simulink model "simscape_earth"  (R2022a)
settings: Solver=ode4  StartTime=0.0  StopTime=12000  FixedStep=1  RelTol=1e-3
undefined symbols (not defined in the file or in its folder): X, Y, Z
libraries: sm_lib x6, nesl_utility x4
settings Model: Creator=sakur  LastModifiedBy=sakur

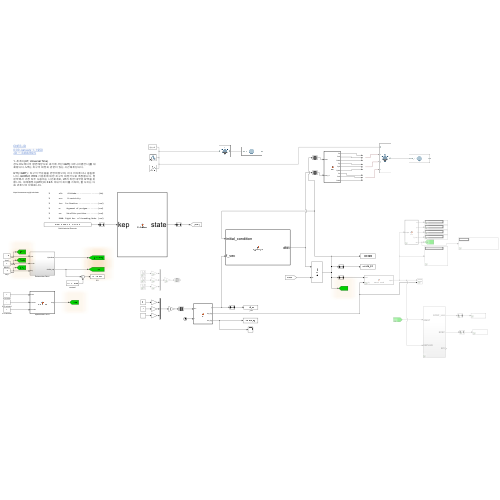
[thumbnail: Simulink's stored preview of the top-level diagram]
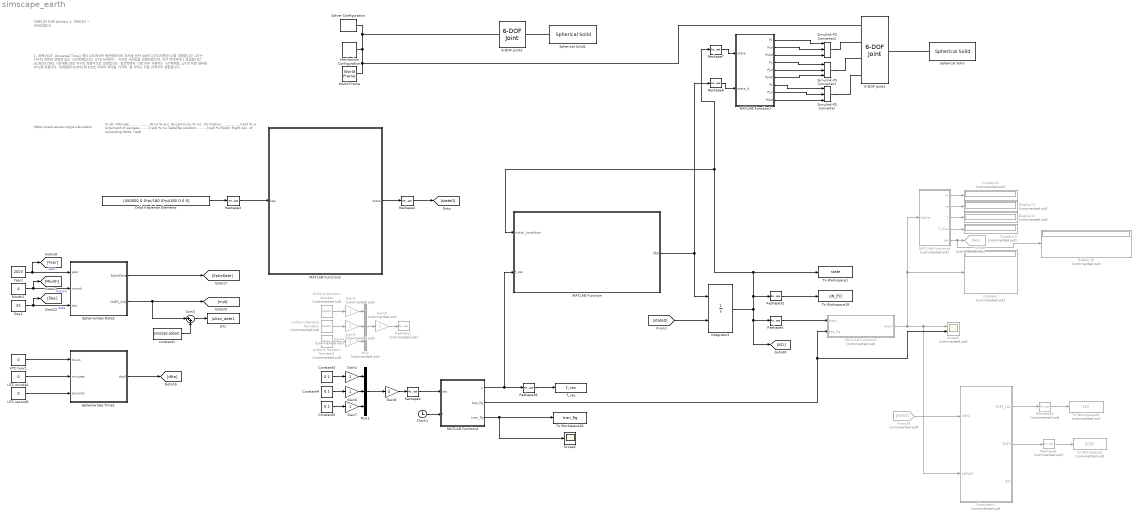
== system simscape_earth ==
  note: % alt: Altitude.....................(Km)
      | % ecc: Eccentricity
      | % inc: Inclination...................(rad)
      | % w: Argument of perigee..........(rad)
      | % nu: Satellite position...........(rad) % RAAN: Right Asc. of Ascending Node. (rad)
  note: 1. 세계시(UT, Universal Time)
      | 경도 0도에서의 평균태양시로 과거에 쓰던 GMT(그리니치평균시)를 대체합니다. UT는 지구의 회전과 관련이 있는 시간체계입니다.
      |
      | UT1(=GMT) : 지구의 극운동을 반영하였으며, 지구 어디에서나 동일합니다. GCRS와 ITRS 기준계에 대한 지구의 회전각으로 측정합니다. 천문학에서 가장 자주 사용하는 시간체계로, UT라 하면 대부분 UT1을 뜻합니다. 세계협정시(UTC)와 0.9초 이내의 차이를 가지며, 둘 사이는 다음 관계식이 성립됩니다.
  note: CNES JD
      | 0:00 January 1, 1950
      | JD − 2433282.5
  note: https://www.aavso.org/jd-calculator
  6-DOF Joint1 : sm_lib/Joints/6-DOF Joint  JointMode=Normal  SenseConstraintForce=off  SenseConstraintForceX=off  SenseConstraintForceY=off  SenseConstraintForceZ=off  SenseConstraintTorque=off  SenseConstraintTorqueX=off  SenseConstraintTorqueY=off  SenseConstraintTorqueZ=off  SenseTotalForce=off  SenseTotalForceX=off  SenseTotalForceY=off  SenseTotalForceZ=off  SenseTotalTorque=off  SenseTotalTorqueX=off  SenseTotalTorqueY=off  SenseTotalTorqueZ=off  CompositeWrenchDir=FollowerOnBase  CompositeWrenchFrame=BaseFrame  PxEquilibriumPosition=0  PxEquilibriumPositionUnits=m  PxSpringStiffness=0  PxSpringStiffnessUnits=N/m  PxDampingCoefficient=0  PxDampingCoefficientUnits=N/(m/s)  PxTorqueActuationMode=ComputedTorque  PxMotionActuationMode=InputMotion  PxSensePosition=off  PxSenseVelocity=off  PxSenseAcceleration=off  PxSenseTorqueForce=off  PxSenseLowerLimitTorqueForce=off  PxSenseUpperLimitTorqueForce=off  PxLowerLimitSpecify=off  PxLowerLimitBound=-1  PxLowerLimitBoundUnits=m  PxLowerLimitStiffness=1e6  PxLowerLimitStiffnessUnits=N/m  PxLowerLimitDamping=1e3  PxLowerLimitDampingUnits=N/(m/s)  PxLowerLimitTransitionRegionWidth=1e-4  PxLowerLimitTransitionRegionWidthUnits=m  PxUpperLimitSpecify=off  PxUpperLimitBound=1  PxUpperLimitBoundUnits=m  PxUpperLimitStiffness=1e6  PxUpperLimitStiffnessUnits=N/m  PxUpperLimitDamping=1e3  PxUpperLimitDampingUnits=N/(m/s)  PxUpperLimitTransitionRegionWidth=1e-4  PxUpperLimitTransitionRegionWidthUnits=m  PxPositionTargetSpecify=off  PxPositionTargetPriority=High  PxPositionTargetValue=0  PxPositionTargetValueUnits=m  PxVelocityTargetSpecify=off  PxVelocityTargetPriority=High  PxVelocityTargetValue=0  PxVelocityTargetValueUnits=m/s  PyEquilibriumPosition=0  PyEquilibriumPositionUnits=m  PySpringStiffness=0  PySpringStiffnessUnits=N/m  PyDampingCoefficient=0  PyDampingCoefficientUnits=N/(m/s)  PyTorqueActuationMode=ComputedTorque  PyMotionActuationMode=InputMotion  PySensePosition=off  PySenseVelocity=off  PySenseAcceleration=off  PySenseTorqueForce=off  PySenseLowerLimitTorqueForce=off  PySenseUpperLimitTorqueForce=off  PyLowerLimitSpecify=off  PyLowerLimitBound=-1  PyLowerLimitBoundUnits=m  PyLowerLimitStiffness=1e6  PyLowerLimitStiffnessUnits=N/m  PyLowerLimitDamping=1e3  PyLowerLimitDampingUnits=N/(m/s)  PyLowerLimitTransitionRegionWidth=1e-4  PyLowerLimitTransitionRegionWidthUnits=m  PyUpperLimitSpecify=off  PyUpperLimitBound=1  PyUpperLimitBoundUnits=m  PyUpperLimitStiffness=1e6  PyUpperLimitStiffnessUnits=N/m  PyUpperLimitDamping=1e3  PyUpperLimitDampingUnits=N/(m/s)  PyUpperLimitTransitionRegionWidth=1e-4  PyUpperLimitTransitionRegionWidthUnits=m  PyPositionTargetSpecify=off  PyPositionTargetPriority=High  PyPositionTargetValue=0  PyPositionTargetValueUnits=m  PyVelocityTargetSpecify=off  PyVelocityTargetPriority=High  PyVelocityTargetValue=0  PyVelocityTargetValueUnits=m/s  PzEquilibriumPosition=0  PzEquilibriumPositionUnits=m  PzSpringStiffness=0  PzSpringStiffnessUnits=N/m  PzDampingCoefficient=0  PzDampingCoefficientUnits=N/(m/s)  PzTorqueActuationMode=ComputedTorque  PzMotionActuationMode=InputMotion  PzSensePosition=off  PzSenseVelocity=off  PzSenseAcceleration=off  PzSenseTorqueForce=off  PzSenseLowerLimitTorqueForce=off  PzSenseUpperLimitTorqueForce=off  PzLowerLimitSpecify=off  PzLowerLimitBound=-1  PzLowerLimitBoundUnits=m  PzLowerLimitStiffness=1e6  PzLowerLimitStiffnessUnits=N/m  PzLowerLimitDamping=1e3  PzLowerLimitDampingUnits=N/(m/s)  PzLowerLimitTransitionRegionWidth=1e-4  PzLowerLimitTransitionRegionWidthUnits=m  PzUpperLimitSpecify=off  PzUpperLimitBound=1  PzUpperLimitBoundUnits=m  PzUpperLimitStiffness=1e6  PzUpperLimitStiffnessUnits=N/m  PzUpperLimitDamping=1e3  PzUpperLimitDampingUnits=N/(m/s)  PzUpperLimitTransitionRegionWidth=1e-4  PzUpperLimitTransitionRegionWidthUnits=m  PzPositionTargetSpecify=off  PzPositionTargetPriority=High  PzPositionTargetValue=0  PzPositionTargetValueUnits=m  PzVelocityTargetSpecify=off  PzVelocityTargetPriority=High  PzVelocityTargetValue=0  PzVelocityTargetValueUnits=m/s  SphDefPosRotationMethod=None  SphDefPosRotationAngleUnits=deg  SphDefPosRotationStandardAxis=+Z  SphDefPosRotationAngle=0.0  SphDefPosRotationArbitraryAxis=[0 0 1]  SphDefPosFollAlignAxisA=+X  SphDefPosBaseAlignAxisA=+Y  SphDefPosFollAlignAxisB=+Y  SphDefPosBaseAlignAxisB=+Z  SphDefPosRotationSequenceAxes=FollowerAxes  SphDefPosRotationSequence=XYX  SphDefPosRotationSequenceAngles=[0 0 0]  SphDefPosRotationSequenceAnglesUnits=deg  SphDefPosRotationMatrix=[1 0 0; 0 1 0; 0 0 1]  SphEqPosRotationMethod=None  SphEqPosRotationAngleUnits=deg  SphEqPosRotationStandardAxis=+Z  SphEqPosRotationAngle=0.0  SphEqPosRotationArbitraryAxis=[0 0 1]  SphEqPosFollAlignAxisA=+X  SphEqPosBaseAlignAxisA=+Y  SphEqPosFollAlignAxisB=+Y  SphEqPosBaseAlignAxisB=+Z  SphEqPosRotationSequenceAxes=FollowerAxes  SphEqPosRotationSequence=XYX  SphEqPosRotationSequenceAngles=[0 0 0]  SphEqPosRotationSequenceAnglesUnits=deg  SphEqPosRotationMatrix=[1 0 0; 0 1 0; 0 0 1]  SphSpringStiffness=0  SphSpringStiffnessUnits=N*m/deg  SphDampingCoefficient=0  SphDampingCoefficientUnits=N*m/(deg/s)  SphActuateTorqueX=off  SphActuateTorqueY=off  SphActuateTorqueZ=off  SphActuateTorque=off  SphTorqueActuationMode=NoTorque  SphMotionActuationMode=ComputedMotion  SphActuationFrame=BaseFrame  SphSensePosition=off  SphSenseVelocityX=off  SphSenseVelocityY=off  SphSenseVelocityZ=off  SphSenseVelocity=off  SphSenseAccelerationX=off  SphSenseAccelerationY=off  SphSenseAccelerationZ=off  SphSenseAcceleration=off  SphSenseTorqueX=off  SphSenseTorqueY=off  SphSenseTorqueZ=off  SphSenseTorqueForce=off  SphSenseLowerLimitTorqueMag=off  SphSenseUpperLimitTorqueMag=off  SphSensingFrame=BaseFrame  SphLowerLimitSpecify=off  SphLowerLimitBound=15  SphLowerLimitBoundUnits=deg  SphLowerLimitStiffness=1e4  SphLowerLimitStiffnessUnits=N*m/deg  SphLowerLimitDamping=10  SphLowerLimitDampingUnits=N*m/(deg/s)  SphLowerLimitTransitionRegionWidth=0.1  SphLowerLimitTransitionRegionWidthUnits=deg  SphUpperLimitSpecify=off  SphUpperLimitBound=45  SphUpperLimitBoundUnits=deg  SphUpperLimitStiffness=1e4  SphUpperLimitStiffnessUnits=N*m/deg  SphUpperLimitDamping=10  SphUpperLimitDampingUnits=N*m/(deg/s)  SphUpperLimitTransitionRegionWidth=0.1  SphUpperLimitTransitionRegionWidthUnits=deg  SphPositionTargetRotationMethod=None  SphPositionTargetRotationAngleUnits=deg  SphPositionTargetRotationStandardAxis=+Z  SphPositionTargetRotationAngle=0.0  SphPositionTargetRotationArbitraryAxis=[0 0 1]  SphPositionTargetFollAlignAxisA=+X  SphPositionTargetBaseAlignAxisA=+Y  SphPositionTargetFollAlignAxisB=+Y  SphPositionTargetBaseAlignAxisB=+Z  SphPositionTargetRotationSequenceAxes=FollowerAxes  SphPositionTargetRotationSequence=XYX  SphPositionTargetRotationSequenceAngles=[0 0 0]  SphPositionTargetRotationSequenceAnglesUnits=deg  SphPositionTargetRotationMatrix=[1 0 0; 0 1 0; 0 0 1]  SphPositionTargetSpecify=off  SphPositionTargetPriority=High  SphVelocityTargetValue=[0 0 0]  SphVelocityTargetValueUnits=deg/s  SphVelocityTargetSpecify=off  SphVelocityTargetPriority=High  SphVelocityTargetInFollowerFrame=on
  6-DOF Joint2 : sm_lib/Joints/6-DOF Joint  JointMode=Normal  SenseConstraintForce=off  SenseConstraintForceX=off  SenseConstraintForceY=off  SenseConstraintForceZ=off  SenseConstraintTorque=off  SenseConstraintTorqueX=off  SenseConstraintTorqueY=off  SenseConstraintTorqueZ=off  SenseTotalForce=off  SenseTotalForceX=off  SenseTotalForceY=off  SenseTotalForceZ=off  SenseTotalTorque=off  SenseTotalTorqueX=off  SenseTotalTorqueY=off  SenseTotalTorqueZ=off  CompositeWrenchDir=FollowerOnBase  CompositeWrenchFrame=BaseFrame  PxEquilibriumPosition=0  PxEquilibriumPositionUnits=m  PxSpringStiffness=0  PxSpringStiffnessUnits=N/m  PxDampingCoefficient=0  PxDampingCoefficientUnits=N/(m/s)  PxTorqueActuationMode=NoTorque  PxMotionActuationMode=ComputedMotion  PxSensePosition=off  PxSenseVelocity=off  PxSenseAcceleration=off  PxSenseTorqueForce=off  PxSenseLowerLimitTorqueForce=off  PxSenseUpperLimitTorqueForce=off  PxLowerLimitSpecify=off  PxLowerLimitBound=-1  PxLowerLimitBoundUnits=m  PxLowerLimitStiffness=1e6  PxLowerLimitStiffnessUnits=N/m  PxLowerLimitDamping=1e3  PxLowerLimitDampingUnits=N/(m/s)  PxLowerLimitTransitionRegionWidth=1e-4  PxLowerLimitTransitionRegionWidthUnits=m  PxUpperLimitSpecify=off  PxUpperLimitBound=1  PxUpperLimitBoundUnits=m  PxUpperLimitStiffness=1e6  PxUpperLimitStiffnessUnits=N/m  PxUpperLimitDamping=1e3  PxUpperLimitDampingUnits=N/(m/s)  PxUpperLimitTransitionRegionWidth=1e-4  PxUpperLimitTransitionRegionWidthUnits=m  PxPositionTargetSpecify=off  PxPositionTargetPriority=High  PxPositionTargetValue=0  PxPositionTargetValueUnits=m  PxVelocityTargetSpecify=off  PxVelocityTargetPriority=High  PxVelocityTargetValue=0  PxVelocityTargetValueUnits=m/s  PyEquilibriumPosition=0  PyEquilibriumPositionUnits=m  PySpringStiffness=0  PySpringStiffnessUnits=N/m  PyDampingCoefficient=0  PyDampingCoefficientUnits=N/(m/s)  PyTorqueActuationMode=NoTorque  PyMotionActuationMode=ComputedMotion  PySensePosition=off  PySenseVelocity=off  PySenseAcceleration=off  PySenseTorqueForce=off  PySenseLowerLimitTorqueForce=off  PySenseUpperLimitTorqueForce=off  PyLowerLimitSpecify=off  PyLowerLimitBound=-1  PyLowerLimitBoundUnits=m  PyLowerLimitStiffness=1e6  PyLowerLimitStiffnessUnits=N/m  PyLowerLimitDamping=1e3  PyLowerLimitDampingUnits=N/(m/s)  PyLowerLimitTransitionRegionWidth=1e-4  PyLowerLimitTransitionRegionWidthUnits=m  PyUpperLimitSpecify=off  PyUpperLimitBound=1  PyUpperLimitBoundUnits=m  PyUpperLimitStiffness=1e6  PyUpperLimitStiffnessUnits=N/m  PyUpperLimitDamping=1e3  PyUpperLimitDampingUnits=N/(m/s)  PyUpperLimitTransitionRegionWidth=1e-4  PyUpperLimitTransitionRegionWidthUnits=m  PyPositionTargetSpecify=off  PyPositionTargetPriority=High  PyPositionTargetValue=0  PyPositionTargetValueUnits=m  PyVelocityTargetSpecify=off  PyVelocityTargetPriority=High  PyVelocityTargetValue=0  PyVelocityTargetValueUnits=m/s  PzEquilibriumPosition=0  PzEquilibriumPositionUnits=m  PzSpringStiffness=0  PzSpringStiffnessUnits=N/m  PzDampingCoefficient=0  PzDampingCoefficientUnits=N/(m/s)  PzTorqueActuationMode=NoTorque  PzMotionActuationMode=ComputedMotion  PzSensePosition=off  PzSenseVelocity=off  PzSenseAcceleration=off  PzSenseTorqueForce=off  PzSenseLowerLimitTorqueForce=off  PzSenseUpperLimitTorqueForce=off  PzLowerLimitSpecify=off  PzLowerLimitBound=-1  PzLowerLimitBoundUnits=m  PzLowerLimitStiffness=1e6  PzLowerLimitStiffnessUnits=N/m  PzLowerLimitDamping=1e3  PzLowerLimitDampingUnits=N/(m/s)  PzLowerLimitTransitionRegionWidth=1e-4  PzLowerLimitTransitionRegionWidthUnits=m  PzUpperLimitSpecify=off  PzUpperLimitBound=1  PzUpperLimitBoundUnits=m  PzUpperLimitStiffness=1e6  PzUpperLimitStiffnessUnits=N/m  PzUpperLimitDamping=1e3  PzUpperLimitDampingUnits=N/(m/s)  PzUpperLimitTransitionRegionWidth=1e-4  PzUpperLimitTransitionRegionWidthUnits=m  PzPositionTargetSpecify=off  PzPositionTargetPriority=High  PzPositionTargetValue=0  PzPositionTargetValueUnits=m  PzVelocityTargetSpecify=off  PzVelocityTargetPriority=High  PzVelocityTargetValue=0  PzVelocityTargetValueUnits=m/s  SphDefPosRotationMethod=None  SphDefPosRotationAngleUnits=deg  SphDefPosRotationStandardAxis=+Z  SphDefPosRotationAngle=0.0  SphDefPosRotationArbitraryAxis=[0 0 1]  SphDefPosFollAlignAxisA=+X  SphDefPosBaseAlignAxisA=+Y  SphDefPosFollAlignAxisB=+Y  SphDefPosBaseAlignAxisB=+Z  SphDefPosRotationSequenceAxes=FollowerAxes  SphDefPosRotationSequence=XYX  SphDefPosRotationSequenceAngles=[0 0 0]  SphDefPosRotationSequenceAnglesUnits=deg  SphDefPosRotationMatrix=[1 0 0; 0 1 0; 0 0 1]  SphEqPosRotationMethod=None  SphEqPosRotationAngleUnits=deg  SphEqPosRotationStandardAxis=+Z  SphEqPosRotationAngle=0.0  SphEqPosRotationArbitraryAxis=[0 0 1]  SphEqPosFollAlignAxisA=+X  SphEqPosBaseAlignAxisA=+Y  SphEqPosFollAlignAxisB=+Y  SphEqPosBaseAlignAxisB=+Z  SphEqPosRotationSequenceAxes=FollowerAxes  SphEqPosRotationSequence=XYX  SphEqPosRotationSequenceAngles=[0 0 0]  SphEqPosRotationSequenceAnglesUnits=deg  SphEqPosRotationMatrix=[1 0 0; 0 1 0; 0 0 1]  SphSpringStiffness=0  SphSpringStiffnessUnits=N*m/deg  SphDampingCoefficient=0  SphDampingCoefficientUnits=N*m/(deg/s)  SphActuateTorqueX=off  SphActuateTorqueY=off  SphActuateTorqueZ=off  SphActuateTorque=off  SphTorqueActuationMode=NoTorque  SphMotionActuationMode=ComputedMotion  SphActuationFrame=BaseFrame  SphSensePosition=off  SphSenseVelocityX=off  SphSenseVelocityY=off  SphSenseVelocityZ=off  SphSenseVelocity=off  SphSenseAccelerationX=off  SphSenseAccelerationY=off  SphSenseAccelerationZ=off  SphSenseAcceleration=off  SphSenseTorqueX=off  SphSenseTorqueY=off  SphSenseTorqueZ=off  SphSenseTorqueForce=off  SphSenseLowerLimitTorqueMag=off  SphSenseUpperLimitTorqueMag=off  SphSensingFrame=BaseFrame  SphLowerLimitSpecify=off  SphLowerLimitBound=15  SphLowerLimitBoundUnits=deg  SphLowerLimitStiffness=1e4  SphLowerLimitStiffnessUnits=N*m/deg  SphLowerLimitDamping=10  SphLowerLimitDampingUnits=N*m/(deg/s)  SphLowerLimitTransitionRegionWidth=0.1  SphLowerLimitTransitionRegionWidthUnits=deg  SphUpperLimitSpecify=off  SphUpperLimitBound=45  SphUpperLimitBoundUnits=deg  SphUpperLimitStiffness=1e4  SphUpperLimitStiffnessUnits=N*m/deg  SphUpperLimitDamping=10  SphUpperLimitDampingUnits=N*m/(deg/s)  SphUpperLimitTransitionRegionWidth=0.1  SphUpperLimitTransitionRegionWidthUnits=deg  SphPositionTargetRotationMethod=None  SphPositionTargetRotationAngleUnits=deg  SphPositionTargetRotationStandardAxis=+Z  SphPositionTargetRotationAngle=0.0  SphPositionTargetRotationArbitraryAxis=[0 0 1]  SphPositionTargetFollAlignAxisA=+X  SphPositionTargetBaseAlignAxisA=+Y  SphPositionTargetFollAlignAxisB=+Y  SphPositionTargetBaseAlignAxisB=+Z  SphPositionTargetRotationSequenceAxes=FollowerAxes  SphPositionTargetRotationSequence=XYX  SphPositionTargetRotationSequenceAngles=[0 0 0]  SphPositionTargetRotationSequenceAnglesUnits=deg  SphPositionTargetRotationMatrix=[1 0 0; 0 1 0; 0 0 1]  SphPositionTargetSpecify=off  SphPositionTargetPriority=High  SphVelocityTargetValue=[0 0 0]  SphVelocityTargetValueUnits=deg/s  SphVelocityTargetSpecify=off  SphVelocityTargetPriority=High  SphVelocityTargetInFollowerFrame=on
  Clock1 : Clock
  Constant3 : Constant  Value=0.1
  Constant4 : Constant  Value=0.1
  Constant5 : Constant  Value=0.1
  Day1 : Constant  Value=25
  Display{1,10..13,19} (6 alike) : Display  Commented=on
  Ephemerides Date1 : Subsystem
  Ephemerides Time1 : MATLAB Function  TreatAsAtomicUnit=on
  From24 : From  Commented=on  GotoTag=GMST
  Gain1 : Gain
  Gain{2..5} (4 alike) : Gain  Commented=on
  Gain6 : Gain
  Gain7 : Gain
  Gain8 : Gain  Gain=0
  Goto8 : Goto  Commented=on  GotoTag=we
  Integrator2 : Integrator  InitialConditionSource=external  InitialCondition=[-7000 0 0 0 -9.175045 0 5233.5]'
  JD1 : ToWorkspace  VariableName=Julian_date1  SampleTime=-1
  MATLAB Function : MATLAB Function  TreatAsAtomicUnit=on
  MATLAB Function1 : MATLAB Function  TreatAsAtomicUnit=on
  MATLAB Function2 : MATLAB Function  TreatAsAtomicUnit=on
  MATLAB Function4 : MATLAB Function  TreatAsAtomicUnit=on
  MATLAB Function5 : MATLAB Function  Commented=on  TreatAsAtomicUnit=on
  MATLAB Function8 : MATLAB Function  Commented=on  TreatAsAtomicUnit=on
  Mechanism Configuration : sm_lib/Utilities/Mechanism Configuration  UniformGravity=None  GravityVector=[0 0 -9.80665]  GravityUnits=m/s^2  LinearizationDelta=0.001  JointModeTransitionNonlinearIterations=2
  Month1 : Constant  Value=4
  Mux : Mux  Commented=on  Inputs=3
  Mux1 : Mux  Inputs=3
  Orbit Keplerian Elements : Constant  Value=[450000 0 0*pi/180 0*pi/180 0 0 0]
  Reshape1 : Reshape  Commented=on  OutputDimensionality=Column vector (2-D)
  Reshape2 : Reshape  OutputDimensionality=Column vector (2-D)
  Reshape{3..5,28,31} (5 alike) : Reshape  OutputDimensionality=Row vector (2-D)
  Reshape32 : Reshape  Commented=on  OutputDimensionality=Row vector (2-D)
  Reshape6 : Reshape  Commented=on  OutputDimensionality=Row vector (2-D)
  Reshape7 : Reshape  OutputDimensionality=Column vector (2-D)
  Reshape8 : Reshape  OutputDimensionality=Column vector (2-D)
  Scope2 : Scope
  Scope5 : Scope  Commented=on  NumInputPorts=2
  Simulink-PS Converter : nesl_utility/Simulink-PS Converter  PhysicalDomain=network_engine_domain  SubClassName=ps_input  LeftPortType=input  RightPortType=output  PseudoPeriodic=off  Frequencies=[]  NoiseDistribution=none  NoiseParameters=[]  Unit=1  AffineConversion=off  FilteringAndDerivatives=provide  SimscapeFilterOrder=1  InputFilterTimeConstant=0.001  UdotUserProvided=2
      settings: SourceProductBaseCode=SS,PW,VE
  Simulink-PS Converter1 : nesl_utility/Simulink-PS Converter  PhysicalDomain=network_engine_domain  SubClassName=ps_input  LeftPortType=input  RightPortType=output  PseudoPeriodic=off  Frequencies=[]  NoiseDistribution=none  NoiseParameters=[]  Unit=1  AffineConversion=off  FilteringAndDerivatives=provide  SimscapeFilterOrder=1  InputFilterTimeConstant=0.001  UdotUserProvided=2
      settings: SourceProductBaseCode=SS,PW,VE
  Simulink-PS Converter2 : nesl_utility/Simulink-PS Converter  PhysicalDomain=network_engine_domain  SubClassName=ps_input  LeftPortType=input  RightPortType=output  PseudoPeriodic=off  Frequencies=[]  NoiseDistribution=none  NoiseParameters=[]  Unit=1  AffineConversion=off  FilteringAndDerivatives=provide  SimscapeFilterOrder=1  InputFilterTimeConstant=0.001  UdotUserProvided=2
      settings: SourceProductBaseCode=SS,PW,VE
  Solver Configuration : nesl_utility/Solver Configuration  PhysicalDomain=network_engine_domain  SubClassName=solver  LeftPortType=input  RightPortType=generic  Tones=[]  Harmonics=[]  SimulateNoise=off  Profile=off  UseLocalSampling=off  EnableSwitchedLinearOptims=on  FrequencyDomain=off  UseCCode=off  RelTol=0.001  AbsTol=0.001  MinStep=1e-09  ToWorkspace=off  RevertToSquareIcSolve=off  NumHomotopyIterations=100  PhasorMode=off  PhasorModeNumHarmonics=1  IndexReductionMethod=DerivativeReplacement  DoDC=off  ResidualTolerance=1e-09  UseLocalSolver=off  LocalSolverChoice=NE_BACKWARD_EULER_ADVANCER  LocalSolverSampleTime=0.001  DoFixedCost=off  MaxNonlinIter=3  MaxModeIter=2  ComputeImpulses=off  ImpulseIterations=2  LinearAlgebra=auto  LinearAlgebraNumThread=0  EquationFormulation=NE_TIME_EF  DelaysMemoryBudget=1024  AutomaticFiltering=on  FilteringTimeConstant=0.001  PartitionStorageMethod=AS_NEEDED  PartitionMemoryBudget=1024  PartitionMethod=ROBUST
      settings: SourceProductBaseCode=SS,PW,VE
  Spherical Solid : sm_lib/Body Elements/Spherical Solid  GraphicAmbientColor=[0.15 0.15 0.15 1.0]  BasedOnType=Mass  CenterOfMass=[0 0 0]  CenterOfMassUnits=m  GraphicDiffuseColor=[1.0 1.0 0.0]  Density=1000  DensityUnits=kg/m^3  DoExposeReferenceFrame=on  GraphicEmissiveColor=[0.0 0.0 0.0 1.0]  ExportEntireGeometry=off  SerializedExposedGeometries=<ExposedGeometries/>  SerializedFrames=<Frames><Frame><Id>Frame1</Id><Value><Name>CoM_F</Name><Origin><Source>CenterOfMassFrame</Source><FeatureName></FeatureName></Origin><PrimaryAxis><DefinedDirection>+Z</DefinedDirection><Source>ReferenceFrame</Source><SourceDirection>+Z</SourceDirection><FeatureName></FeatureName></PrimaryAxis><SecondaryAxis><DefinedDirection>+X</DefinedDirection><Source>ReferenceFrame</Source><SourceDirection>+X</SourceDirection><FeatureName></FeatureName></SecondaryAxis></Value></Frame></Frames>  MarkerShape=Sphere  MarkerSize=10  GraphicType=FromGeometry  InertiaType=CalculateFromGeometry  Mass=5.972*(10^24)  MassUnits=kg  MomentsOfInertia=[1 1 1]  MomentsOfInertiaUnits=kg*m^2  GraphicOpacity=1.0  ProductsOfInertia=[0 0 0]  ProductsOfInertiaUnits=kg*m^2  GraphicShininess=75  GraphicSpecularColor=[0.5 0.5 0.5 1.0]  SphereRadius=100000  SphereRadiusUnits=m  GraphicVisPropType=SimpleVisualProperties
  Spherical Solid1 : sm_lib/Body Elements/Spherical Solid  GraphicAmbientColor=[0.15 0.15 0.15 1.0]  BasedOnType=Mass  CenterOfMass=[0 0 0]  CenterOfMassUnits=m  GraphicDiffuseColor=[0.0 0.6 0.6]  Density=1000  DensityUnits=kg/m^3  DoExposeReferenceFrame=on  GraphicEmissiveColor=[0.0 0.0 0.0 1.0]  ExportEntireGeometry=off  SerializedExposedGeometries=<ExposedGeometries/>  SerializedFrames=<Frames><Frame><Id>Frame1</Id><Value><Name>CoM_F</Name><Origin><Source>CenterOfMassFrame</Source><FeatureName></FeatureName></Origin><PrimaryAxis><DefinedDirection>+Z</DefinedDirection><Source>ReferenceFrame</Source><SourceDirection>+Z</SourceDirection><FeatureName></FeatureName></PrimaryAxis><SecondaryAxis><DefinedDirection>+X</DefinedDirection><Source>ReferenceFrame</Source><SourceDirection>+X</SourceDirection><FeatureName></FeatureName></SecondaryAxis></Value></Frame></Frames>  MarkerShape=Sphere  MarkerSize=10  GraphicType=FromGeometry  InertiaType=CalculateFromGeometry  Mass=5.972*(10^24)  MassUnits=kg  MomentsOfInertia=[1 1 1]  MomentsOfInertiaUnits=kg*m^2  GraphicOpacity=1.0  ProductsOfInertia=[0 0 0]  ProductsOfInertiaUnits=kg*m^2  GraphicShininess=75  GraphicSpecularColor=[0.5 0.5 0.5 1.0]  SphereRadius=6371000  SphereRadiusUnits=m  GraphicVisPropType=AdvancedVisualProperties
  Subsystem1 : Subsystem  Commented=on
  Sum2 : Sum  Inputs=|++
  To Workspace1 : ToWorkspace  VariableName=state  SampleTime=-1
      settings: Save2DSignal=2-D array (concatenate along first dimension)
  To Workspace18 : ToWorkspace  VariableName=tran_flg  SampleTime=-1
      settings: Save2DSignal=2-D array (concatenate along first dimension)
  To Workspace19 : ToWorkspace  VariableName=LIN_ECI  SampleTime=-1
      settings: Save2DSignal=2-D array (concatenate along first dimension)
  To Workspace2 : ToWorkspace  Commented=on  VariableName=ECEF  SampleTime=-1
      settings: Save2DSignal=2-D array (concatenate along first dimension)
  To Workspace20 : ToWorkspace  Commented=on  VariableName=LLA  SampleTime=-1
      settings: Save2DSignal=2-D array (concatenate along first dimension)
  UTC hour1 : Constant  Value=0
  UTC minute1 : Constant  Value=0
  UTC second1 : Constant  Value=0
  Uniform Random Number : UniformRandomNumber  Commented=on  Minimum=-0.5  Maximum=0.5  SampleTime=1
  Uniform Random Number1 : UniformRandomNumber  Commented=on  Minimum=-0.5  Maximum=0.5  SampleTime=1
  Uniform Random Number2 : UniformRandomNumber  Commented=on  Minimum=-0.5  Maximum=0.5  SampleTime=1
  World Frame : sm_lib/Frames and Transforms/World Frame
  Year1 : Constant  Value=2023
  constant1 : Constant  Value=2433282.50000
  f_vec : ToWorkspace  VariableName=f_vec  SampleTime=-1
      settings: Save2DSignal=2-D array (concatenate along first dimension)
  wires:
  Ephemerides Time1/1(dayf) -> [dfra]
  MATLAB Function8/1(ra) -> Display10/1
  Gain8/1 -> Reshape2/1
  MATLAB Function8/3(T) -> Display12/1
  Gain2/1 -> Mux/1
  Reshape28/1 -> f_vec/1
  Orbit Keplerian Elements/1 -> Reshape3/1
  Gain1/1 -> Mux1/1
  UTC second1/1 -> Ephemerides Time1/3(seconds)
  Year1/1 -> Ephemerides Date1/1(year), [Year]  "year"
  MATLAB Function8/2(rp) -> Display11/1
  UTC hour1/1 -> Ephemerides Time1/1(hours)
  MATLAB Function8/4(T_hour) -> Display13/1
  Sum2/1 -> JD1/1
  Gain7/1 -> Mux1/3
  MATLAB Function4/1(y) -> MATLAB Function/2(f_vec), Reshape28/1
  Month1/1 -> [Month], Ephemerides Date1/2(month)  "month"
  Mux1/1 -> Gain8/1
  Clock1/1 -> MATLAB Function4/2(t)
  Gain6/1 -> Mux1/2
  Ephemerides Date1/2(CNES_mdj) -> Sum2/1, [mjd]
  Reshape5/1 -> MATLAB Function5/1(statv)
  Mux/1 -> Gain5/1
  MATLAB Function5/1(kepel) -> MATLAB Function8/1(kepler), Display1/1, Subsystem1/2(KEPLER), Scope5/1
  Uniform Random Number/1 -> Gain2/1
  Uniform Random Number1/1 -> Gain3/1
  MATLAB Function4/3(tran_flg) -> Scope2/1, To Workspace18/1
  Constant5/1 -> Gain7/1
  MATLAB Function2/1(state) -> Reshape4/1
  [state0] -> Integrator2/2
  MATLAB Function/1(dfdt) -> Integrator2/1, Reshape8/1
  Ephemerides Date1/1(EpheDate) -> [EpheDate]
  Reshape3/1 -> MATLAB Function2/1(kep)
  Reshape6/1 -> To Workspace2/1
  Constant3/1 -> Gain1/1
  Reshape31/1 -> To Workspace19/1
  Reshape4/1 -> [state0]
  MATLAB Function4/2(kep_flg) -> Scope5/2, MATLAB Function5/2(kep_flg)
  Uniform Random Number2/1 -> Gain4/1
  UTC minute1/1 -> Ephemerides Time1/2(minutes)
  Gain4/1 -> Mux/3
  Day1/1 -> [Day], Ephemerides Date1/3(day)  "date"
  Gain5/1 -> Reshape1/1
  Subsystem1/2(ECEF) -> Reshape6/1
  constant1/1 -> Sum2/2
  MATLAB Function8/5(we) -> Display19/1, Goto8/1
  From24/1 -> Subsystem1/1(GMST)
  Gain3/1 -> Mux/2
  Reshape2/1 -> MATLAB Function4/1(vec)
  Constant4/1 -> Gain6/1
  Reshape32/1 -> To Workspace20/1
  Subsystem1/1(ECEF_LLA) -> Reshape32/1
  Integrator2/1 -> MATLAB Function/1(initial_condition), Reshape7/1, To Workspace1/1, Reshape31/1, Reshape5/1, [ECI]
  MATLAB Function1/7(Pz) -> Simulink-PS Converter/1
  MATLAB Function1/4(Py) -> Simulink-PS Converter1/1
  MATLAB Function1/1(Px) -> Simulink-PS Converter2/1
  Reshape7/1 -> MATLAB Function1/1(state)
  Reshape8/1 -> MATLAB Function1/2(state_d)
  MATLAB Function1/2(Pxd) -> Simulink-PS Converter2/2
  MATLAB Function1/3(Pxdd) -> Simulink-PS Converter2/3
  MATLAB Function1/5(Pyd) -> Simulink-PS Converter1/2
  MATLAB Function1/6(Pydd) -> Simulink-PS Converter1/3
  MATLAB Function1/8(Pzd) -> Simulink-PS Converter/2
  MATLAB Function1/9(Pzdd) -> Simulink-PS Converter/3
  connections:
  Solver Configuration/RConn1 -- Mechanism Configuration/RConn1 -- 6-DOF Joint1/LConn1 -- World Frame/RConn1 -- 6-DOF Joint2/LConn1
  Spherical Solid/LConn1 -- 6-DOF Joint1/RConn1
  Simulink-PS Converter/RConn1 -- 6-DOF Joint1/LConn4
  Simulink-PS Converter1/RConn1 -- 6-DOF Joint1/LConn3
  Simulink-PS Converter2/RConn1 -- 6-DOF Joint1/LConn2
  Spherical Solid1/LConn1 -- 6-DOF Joint2/RConn1

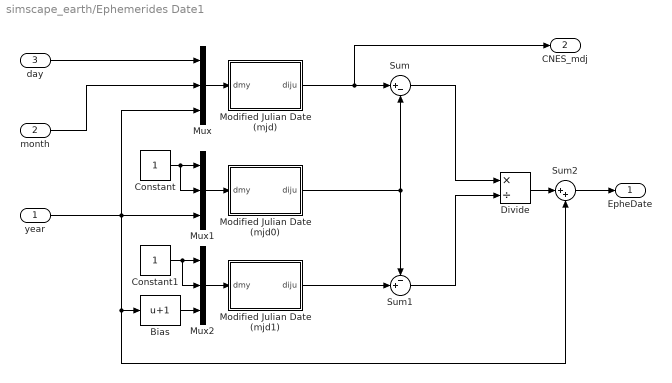
== system simscape_earth/Ephemerides Date1 ==
  year : Inport
  month : Inport  Port=2
  day : Inport  Port=3
  Bias : Bias  Bias=1  SaturateOnIntegerOverflow=off
  Constant : Constant
  Constant1 : Constant
  Divide : Product  Inputs=*/
  Modified Julian Date (mjd) : MATLAB Function  TreatAsAtomicUnit=on
  Modified Julian Date (mjd0) : MATLAB Function  TreatAsAtomicUnit=on
  Modified Julian Date (mjd1) : MATLAB Function  TreatAsAtomicUnit=on
  Mux : Mux  Inputs=3
  Mux1 : Mux  Inputs=3
  Mux2 : Mux  Inputs=3
  Sum : Sum  Inputs=|+-
  Sum1 : Sum  Inputs=-+|
  Sum2 : Sum  Inputs=|++
  EpheDate : Outport
  CNES_mdj : Outport  Port=2
  wires:
  Sum1/1 -> Divide/2
  Modified Julian Date (mjd1)/1(diju) -> Sum1/2
  month/1 -> Mux/2
  year/1 -> Mux1/3, Mux/3, Bias/1, Sum2/2
  Mux1/1 -> Modified Julian Date (mjd0)/1(dmy)
  day/1 -> Mux/1
  Mux/1 -> Modified Julian Date (mjd)/1(dmy)
  Mux2/1 -> Modified Julian Date (mjd1)/1(dmy)
  Bias/1 -> Mux2/3
  Modified Julian Date (mjd)/1(diju) -> CNES_mdj/1, Sum/1
  Constant1/1 -> Mux2/2, Mux2/1
  Sum/1 -> Divide/1
  Constant/1 -> Mux1/2, Mux1/1
  Modified Julian Date (mjd0)/1(diju) -> Sum1/1, Sum/2
  Divide/1 -> Sum2/1
  Sum2/1 -> EpheDate/1

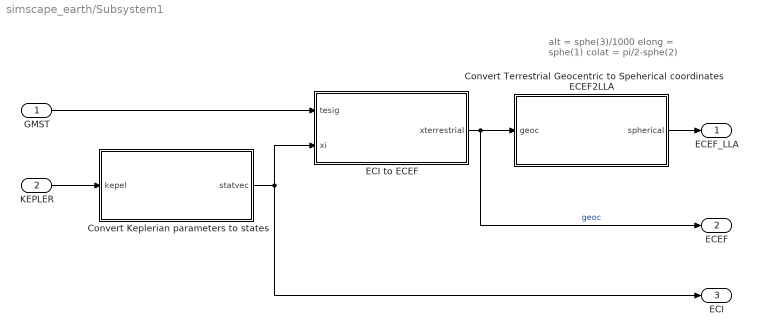
== system simscape_earth/Subsystem1 ==
  note: alt = sphe(3)/1000
      | elong = sphe(1)
      | colat = pi/2-sphe(2)
  GMST : Inport
  KEPLER : Inport  Port=2
  Convert Keplerian parameters to states : MATLAB Function  TreatAsAtomicUnit=on
  Convert Terrestrial Geocentric to Speherical coordinates ECEF2LLA : MATLAB Function  TreatAsAtomicUnit=on
  "ECI to ECEF " : MATLAB Function  TreatAsAtomicUnit=on
  ECEF_LLA : Outport
  ECEF : Outport  Port=2
  ECI : Outport  Port=3
  wires:
  "ECI to ECEF "/1(xterrestrial) -> ECEF/1, Convert Terrestrial Geocentric to Speherical coordinates ECEF2LLA/1(geoc)  "geoc"
  Convert Terrestrial Geocentric to Speherical coordinates ECEF2LLA/1(spherical) -> ECEF_LLA/1
  Convert Keplerian parameters to states/1(statvec) -> "ECI to ECEF "/2(xi), ECI/1
  GMST/1 -> "ECI to ECEF "/1(tesig)
  KEPLER/1 -> Convert Keplerian parameters to states/1(kepel)

== matlab function simscape_earth/Subsystem1/Convert Keplerian parameters to states ==
  data: kepel input; statvec output
function statvec = kepel_statvec(kepel)
%  [statvec] = kepel_statvec (kepel)
%	The function kepel_statvec transforms the keplerian
%	elements kepel into the corresponding state vector in
%	the same reference system.
%
% Input:
%	kepel
% 		vector containing the keplerian elements:
%		(1) - semimajor axis of the orbit in meters.
%		(2) - eccentricity.
%		(3) - inclination in radians.
%		(4) - right ascension of ascending node in radians.
%		(5) - argument of perigee in radians.
%		(6) - mean anomaly in radians.
%
% Output:
%	statvec
%  		state vector in meters and meters/second.
%
% Authors:
%	Helio K. Kuga;
%	Valder M. Medeiros;
%	Valdemir Carrara		february/80		version 1.0
%	Valdemir Carrara		july 2005		(C version)
%   Valdemir Carrara            March/09        Matlab

EARTH_GRAVITY	= 3.9860064e+14;		% Earth's gravitational constant (m**3/s**2)

a    = kepel(1);	% semi-major axis
exc  = kepel(2);	% eccentricity

c1   = sqrt(1. - exc*exc);

% Rotational matrix
rot_maz1 =  [cos(-kepel(4)), sin(-kepel(4)), 0;
             -sin(-kepel(4)), cos(-kepel(4)), 0; 
             0, 0, 1];
         
rot_max =  [1, 0, 0; 
           0, cos(-kepel(3)), sin(-kepel(3));
           0, -sin(-kepel(3)), cos(-kepel(3))];
       
rot_maz2 =  [cos(-kepel(5)), sin(-kepel(5)), 0;
             -sin(-kepel(5)), cos(-kepel(5)), 0; 
             0, 0, 1];
         
orb2iner = rot_maz1*rot_max*rot_maz2;

%%%%%%%%%%%%%%%%%%%%%%%%%%%%%%%%%%%%%%%%%%%%
%     Kepler's equation
%E    = kepler(kepel(6), exc);
mean_anomaly = kepel(6);
eccentricity = exc;
%function [eccentric] = kepler (mean_anomaly, eccentricity)
% [eccentric] = kepler (mean_anomaly, eccentricity)
%	The subroutine kepler finds a solution to the
%	kepler's equation.
%
% Input:
%	mean_anomaly
%		mean anomaly in radians.
%	eccentricity
%		eccentricity.
%
% Output:
%	eccentric
%		eccentric anomaly in radians.
%
% Authors:
%	Valder M. de Medeiros		june/81		version 2.0
%	Valdemir Carrara			july 2005	(C version)
%   Valdemir Carrara            March/09        Matlab

exc2    = eccentricity*eccentricity;
am1     = mod (mean_anomaly, 2*pi);
am2     = am1 + am1;
am3     = am1 + am2;
shoot   = am1 + eccentricity*(1. - 0.125*exc2)*sin(am1) + ...
		0.5*exc2*(sin(am2) + 0.75*eccentricity*sin(am3));
shoot   = mod (shoot, 2*pi);

e1      = 1.0;
ic      = 0;

while ((abs(e1) > 1.e-12) && (ic <= 10)) 
	e1    = (shoot - am1 - eccentricity*sin(shoot)) / ...
			(1.0 - eccentricity*cos(shoot));
    shoot = shoot - e1;
    ic    = ic + 1;
end

if (ic >= 10)
    disp ('warning ** subroutine kepler did not converge in 10 iterations');
end

%eccentric = shoot;
E = shoot;
%%%%%%%%%%%%%%%%%%%%%%%%%%%%%%%%%%%%%%%%%%%%%%
sE   = sin(E);
cE   = cos(E);
c3   = sqrt(EARTH_GRAVITY/a)/(1. - exc*cE);

%     state vector

statvec = [[a*(cE - exc), a*c1*sE, 0]*orb2iner', [-c3*sE, c1*c3*cE, 0]*orb2iner'];

== matlab function simscape_earth/Subsystem1/Convert Terrestrial Geocentric to Speherical coordinates ECEF2LLA ==
  data: geoc input; spherical output
function spherical  = rectangular_to_spherical (geoc)
% [spherical] = rectangular_to_spherical (geoc)
%	Function to transform rectangular terrestrial
%	geocentric coordinates in spherical coordinates
%	(longitude, geocentric latitude and distance).
%
% Inputs:
%   geoc
%   		geocentric rectangular coordinates vector in meters
%           (1) geocentric position x (m)
%           (2) geocentric position y (m)
%           (3) geocentric position z (m)
%
% Outputs:
%	spherical
%		Geocentric coordinates vector:
%			1 = east longitude (rad)
%			2 = geocentric latitude (rad)
%			3 = geocentric distance (meters)
%
% Authors:
%   Valdemir Carrara            May/09        Matlab

px = geoc(1);
py = geoc(2);
pz = geoc(3);
ws = px*px + py*py;
rw = sqrt(ws + pz *pz);
lg = atan2(py, px);
lt = atan2(pz, sqrt(ws));
spherical = [lg, lt, rw];

== matlab function simscape_earth/Subsystem1/ECI to ECEF  ==
  data: tesig input; xterrestrial output; xi input
function xterrestrial  = inertial_to_terrestrial (tesig, xi)
% [xterrestrial] = inertial_to_terrestrial (tesig, xi)
%	The function inertial_to_terrestrial transforms geocentric
%	inertial state vector into geocentric
%	terrestrial coordinates (referred to
%	Greenwich).
%
% Input:
%	tesig
%		Greenwich sidereal time in radians.
%	xi
%		geocentric inertial position vector.
%       (1) inertial geocentric position x (m)
%       (2) inertial geocentric position y (m)
%       (3) inertial geocentric position z (m)
%       (4) inertial geocentric velocity x (m/s)
%       (5) inertial geocentric velocity y (m/s)
%       (6) inertial geocentric velocity z (m/s)
%
% Output:
%	xterrestrial
%		corresponding geocentric terrestrial vector.
%
% Authors:
%	Helio/Valder/Valdemir-aug. 1981 - version 1.0
%	Helio		-july 1989 - version 1.1
%	Valdemir Carrara		july 2005		(C version)
%   Valdemir Carrara            March/09        Matlab
coan    =  cos(tesig);
sian    =  sin(tesig);
rot_mat =  [ coan, sian, 0 ;
            -sian, coan, 0 ; 
                0,    0, 1];

xterrestrial_ = [xi(1:3); xi(4:6)]*rot_mat';
xterrestrial  = [xterrestrial_(1,:) xterrestrial_(2,:)];

== matlab function simscape_earth/MATLAB Function1 ==
  data: state input; Px output; Pxd output; Pxdd output; state_d input; Py output; Pyd output; Pydd output; Pz output; Pzd output; Pzdd output
function [Px,Pxd,Pxdd,Py,Pyd,Pydd,Pz,Pzd,Pzdd] = fcn(state, state_d)
Px   = state(1,1);
Py   = state(2,1);
Pz   = state(3,1);
Pxd  = state(4,1);
Pyd  = state(5,1);
Pzd  = state(6,1);
Pxdd = state_d(4,1);
Pydd = state_d(5,1);
Pzdd = state_d(6,1);
end

== matlab function simscape_earth/MATLAB Function ==
  data: initial_condition input; dfdt output; f_vec input
function dfdt  = eq_propagate(initial_condition, f_vec)
% u=3.9865*10^14;
u=3.9865*10^14;
% Re=6378.14;         % Earth Radius
Re = 6378137; % earth radius in m

dfdt = zeros(size(initial_condition));

%x=x
%x1=dx/dt
%dx1/dt = d^2(x)/dt
% f_vec = [rand(1)*0 rand(1)*0 rand(1)*0]';

x1 = initial_condition(4); % x1 = dx/dt
y1 = initial_condition(5); % y1 = dy/dt
z1 = initial_condition(6); % z1 = dz/dt
x  = initial_condition(1); % x
y  = initial_condition(2); % y
z  = initial_condition(3); % z

m  = initial_condition(7); % mass

r=sqrt(x^2+y^2+z^2);

% % %   Keplar Motion Equatnion
% % %  => r_dd + u/(r^3)r_ = 0 => r_dd = -u/(r^3)r_
dfdt(1) = x1;
dfdt(2) = y1;
dfdt(3) = z1;
dfdt(4) = -u*x/r^3 + f_vec(1,1);
dfdt(5) = -u*y/r^3 + f_vec(2,1);
dfdt(6) = -u*z/r^3 + f_vec(3,1);
dfdt(7) = 0;
end

== matlab function simscape_earth/MATLAB Function2 ==
  data: kep input; state output
% function [X, Y, Z, Vx, Vy, Vz] = Kepler2Carts(alt, ecc, inc, w, nu, RAAN)
function state = Kepler2Carts(kep)
%--------------------------------------------------------------------------------------------------------%
%
% 			USAGE: Conversion of Keplerian Classic Orbital Elements into geocentric-equatorial reference system OXYZ
%
% 			AUTHOR: Thameur Chebbi(PhD)		E-MAIL: chebbythamer@gmail.com
%
% 			DATE: 01,Oct,2020
%
% 			DESCIPTION:      This function is created to convert the classical 
%               		     orbital elements to cartesian position and velocity 
%		       		         parameters of any satellite orbit in the geocentric-equatorial
%                            reference system.
%
% 			INPUT:
%           kep0 =>
% 			alt:    Altitude.....................(Km)							
% 			ecc:    Eccentricity											    
% 			inc:	Inclination..................(rad)							
% 			w:	    Argument of perigee..........(rad)	
% 			nu:	    Satellite position...........(rad)							
% 			RAAN:	Right Asc. of Ascending Node.(rad)							
%
% 			OUTPUT:
%			Position Components: 		
% 			[X  Y  Z ]....(Km)
%
%			Velocity Components:
% 			[Vx Vy Vz]....(Km/s) 														
%
alt  = kep(1,1);    ecc  = kep(1,2);
inc  = kep(1,3);    w    = kep(1,4);
nu   = kep(1,5);    RAAN = kep(1,6);
%%---------------------------- Constants ----------------------------------------------%
% mu_earth = 3.986 * 10^5; % Earth Gravitational Constant
mu_earth = 3.9865 * 10^14; % Earth Gravitational Constant
% re = 6378.1; % earth radius in km
re = 6378137; % earth radius in m
%
%%--------------------------------------------------------------------------------------
a = alt + re;
p = a*(1-ecc ^2);
r_0 = p / (1 + ecc * cos(nu));
%
%%--------------- Coordinates in the perifocal reference system Oxyz -----------------%
%
% position vector coordinates
x = r_0 * cos(nu);
y = r_0 * sin(nu);
%
%
% velocity vector coordinates
Vx_ = -(mu_earth/p)^(1/2) * sin(nu);
Vy_ = (mu_earth/p)^(1/2) * (ecc + cos(nu));
%
%
%%-------------- the geocentric-equatorial reference system OXYZ ---------------------%
%
% position vector components X, Y, and Z
X = (cos(RAAN) * cos(w) - sin(RAAN) * sin(w) * cos(inc)) * x + (-cos(RAAN) * sin(w) - sin(RAAN) * cos(w) * cos(inc)) * y;
Y = (sin(RAAN) * cos(w) + cos(RAAN) * sin(w) * cos(inc)) * x + (-sin(RAAN) * sin(w) + cos(RAAN) * cos(w) * cos(inc)) * y;
Z = (sin(w) * sin(inc)) * x + (cos(w) * sin(inc)) * y;
% velocity vector components X', Y', and Z'
Vx = (cos(RAAN) * cos(w) - sin(RAAN) * sin(w) * cos(inc)) * Vx_ + (-cos(RAAN) * sin(w) - sin(RAAN) * cos(w) * cos(inc)) * Vy_;
Vy = (sin(RAAN) * cos(w) + cos(RAAN) * sin(w) * cos(inc)) * Vx_ + (-sin(RAAN) * sin(w) + cos(RAAN) * cos(w) * cos(inc)) * Vy_;
Vz = (sin(w) * sin(inc)) * Vx_ + (cos(w) * sin(inc)) * Vy_;

state = [X,Y,Z,Vx,Vy,Vz,10];

end

== matlab function simscape_earth/MATLAB Function4 ==
  settings: updateMethod=DISCRETE
  data: vec input; y output; kep_flg output; t input; tran_flg output
function [y, kep_flg, tran_flg] = fcn(vec, t)
ft = 10000;
dt = 1000;


persistent first_flg
persistent tran_flg_save


if isempty(first_flg)
    tran_flg_save = 0;
    first_flg = 1;
end

if tran_flg_save == 0
    if( t <= ft )
        y = 0*vec;
    else
        tran_flg_save = tran_flg_save + 1;
        y = 0*vec;
    end
    kep_flg  = 1;

elseif tran_flg_save == 1
    if ((t>ft) && (t<=(ft+dt)))%firing
        y = 1*vec;
        kep_flg  = 0;
    else
        y = 0*vec;
        kep_flg  = 1;
        tran_flg_save = tran_flg_save + 1;
    end

elseif tran_flg_save == 2
    y = 0*vec;
    kep_flg  = 1;
else
    y = 0*vec;
    kep_flg  = 1;
end

tran_flg = tran_flg_save;

% if ((t>=ft) && (t<=(ft+dt)))
%     y = 1*vec;
%     kep_flg  = 0;
%     tran_flg = 1;
% else
%     y = 0*vec;
%     kep_flg  = 1;
%     tran_flg_save = 0;
% end

end

== matlab function simscape_earth/MATLAB Function5 ==
  settings: updateMethod=DISCRETE
  data: statv input; kepel output; kep_flg input
function kepel  = statvec_kepel (statv, kep_flg)
%	The function statvec_kepel transforms the state vector statv
%	into the corresponding keplerian elements in the
%	same reference system.
%
% Input:
%	statv
%		state vector in meters and meters/second.
%
% Output:
%	statvec_kepel
%		vector containing the keplerian elements:
%		(1) - semimajor axis of the orbit in meters.
%		(2) - eccentricity.
%		(3) - inclination in radians.
%		(4) - right ascension of ascending node in radians.
%		(5) - argument of perigee in radians.
%		(6) - mean anomaly in radians.
persistent kepel_save
persistent first_flg

if isempty(first_flg)
    kepel_save = [0 0 0 0 0 0];
    first_flg = 1;
end

EARTH_GRAVITY	= 3.9860064e+14;		% Earth's gravitational constant (m**3/s**2)

if kep_flg == 1
    xp     = [statv(1),statv(2),statv(3)];
    xv     = [statv(4),statv(5),statv(6)];
    r      = sqrt(xp*xp');
    vq     = xv*xv';
    ainv   = 2.0/(r) - vq/EARTH_GRAVITY;

    h      = cross(xp, xv);
    hm     = sqrt(h*h');
    if (hm < 1.e-10)
        disp (' *** Message from function statvec_kepel: *** ');
        disp (' There are no keplerian elements corresponding to this state vector');
        kepel = [0, 0, 0, 0, 0, 0];
    else
        h      = h/hm;
        incl   = acos(h(3));
        raan   = atan2(h(1), -h(2));
        d      = xp*xv' / EARTH_GRAVITY;
        esene  = d * sqrt(EARTH_GRAVITY*ainv);
        ecose  = 1 - r*ainv;
        exc    = sqrt(esene*esene + ecose*ecose);
        E      = atan2(esene, ecose);
        mean   = mod (E - esene, 2*pi);
        an = [0 0 0];
        if mean < 0
            mean = mean + 2*pi;
        end
        if exc < 1.e-10
            arpe = 0;
        else
            dp     = 1./r - ainv;
            ev     = dp*xp - d*xv;
            abev   = sqrt(ev*ev');
            ev     = ev/abev;
            an(1)  = cos(raan);
            an(2)  = sin(raan);
            an(3)  = 0;
            fi     = ev*cross(h, an)';
            arpe = acos(ev*an');
            if fi < 0
                arpe  =  -arpe + 2*pi;
            end
        end

        kepel = [(1./ainv), exc, incl, raan, arpe, mean];
        kepel_save = kepel;
%         T = 2*pi*sqrt((a*a*a)/(EARTH_GRAVITY));
    end
else

    kepel = kepel_save;
    T = 0;
end


end

== matlab function simscape_earth/Ephemerides Date1/Modified Julian Date (mjd) ==
  data: dmy input; diju output
function diju  =  djm (dmy)
% [diju] = djm (day, month, year)
%    The function djm furnishes the Modified Julian
%    Date with reference to the day, month and year,
%    at zero hours of the day.
% inputs:
%   dmy(1): day, day of the month
%   dmy(2): month, month of the year
%   dmy(3): year

% outputs:
%   diju
%       Modified Julian Date in days, referred to 1950.0. 
%
% Valdemir Carrara, Apr, 2003
%

diju = 367*dmy(3) + dmy(1) - 712269 + fix(275*dmy(2)/9)- fix(7*(dmy(3)+fix((dmy(2)+9)/12))/4);

== matlab function simscape_earth/Ephemerides Date1/Modified Julian Date (mjd0) ==
  data: dmy input; diju output
function diju  =  djm (dmy)
% [diju] = djm (day, month, year)
%    The function djm furnishes the Modified Julian
%    Date with reference to the day, month and year,
%    at zero hours of the day.
% inputs:
%   dmy(1): day, day of the month
%   dmy(2): month, month of the year
%   dmy(3): year

% outputs:
%   diju
%       Modified Julian Date in days, referred to 1950.0. 
%
% Valdemir Carrara, Apr, 2003
%

diju = 367*dmy(3) + dmy(1) - 712269 + fix(275*dmy(2)/9)- fix(7*(dmy(3)+fix((dmy(2)+9)/12))/4);

== matlab function simscape_earth/Ephemerides Date1/Modified Julian Date (mjd1) ==
  data: dmy input; diju output
function diju  =  djm (dmy)
% [diju] = djm (day, month, year)
%    The function djm furnishes the Modified Julian
%    Date with reference to the day, month and year,
%    at zero hours of the day.
% inputs:
%   dmy(1): day, day of the month
%   dmy(2): month, month of the year
%   dmy(3): year

% outputs:
%   diju
%       Modified Julian Date in days, referred to 1950.0. 
%
% Valdemir Carrara, Apr, 2003
%

diju = 367*dmy(3) + dmy(1) - 712269 + fix(275*dmy(2)/9)- fix(7*(dmy(3)+fix((dmy(2)+9)/12))/4);

== matlab function simscape_earth/Ephemerides Time1 ==
  data: hours input; dayf output; minutes input; seconds input
function dayf  = time_to_dayf(hours, minutes, seconds)
% [dayf] = time_to_dayf (hours, minutes, seconds)
%    The function time_to_dayf returns with the day elapesed
%    time in seconds
% inputs:
%   hours     
%       day hour (integer).
%   minutes
%       minutes (integer).
%   seconds
%       seconds and fraction of second
% outputs:
%   dayf
%       Day elapsed time in seconds. 
%
% Valdemir Carrara, Feb, 2009
%

dayf = seconds + 60*(minutes + 60*hours);

== matlab function simscape_earth/MATLAB Function8 ==
  data: kepler input; ra output; rp output; T output; T_hour output; we output
function [ra, rp, T, T_hour, we] = fcn(kepler)

u=3.9865*10^14;

a = kepler(1);
e = kepler(2);
% 

ra = a*(1+e);%장반경
rp = a*(1-e);%단반경

a = (ra+rp)/2;

% a = (550 + 6371.8)*1000;

T = 2*pi*sqrt((a*a*a)/(u));

T_hour = T/3600;

we = 2*pi/T;
% we = 1.1207*0.001;

end
